simulink library "pixhawk_slib_sensors_actuators"  (R2017b)
settings: Solver=ode45  StartTime=0.0  StopTime=10.0  RelTol=1e-3
undefined symbols (not defined in the file): PixhawkBlock_InitFcn
libraries: pixhawk_slib_uORB_RW x6
settings Model: Creator=skuznick  LastModifiedBy=uavcs
settings DataIOCC: LimitDataPoints=on  SaveFormat=Array
settings OptimizationCC: BlockReduction=off  BooleanDataType=off  LifeSpan=inf
settings DebuggingCC: SaveWithParameterizedLinksMsg=none  UnderspecifiedInitializationDetection=Classic  MergeDetectMultiDrivingBlocksExec=none  SignalResolutionControl=TryResolveAllWithWarning  AllowSymbolicDim=off  StrictBusMsg=Warning  SFUnexpectedBacktrackingDiag=warning  SFNoUnconditionalDefaultTransitionDiag=warning  SFExecutionAtInitializationDiag=none
settings HardwareCC: ProdBitPerPointer=32  ProdBitPerSizeT=32  ProdBitPerPtrDiffT=32  ProdLargestAtomicFloat=None  ProdIntDivRoundTo=Undefined  ProdEndianess=Unspecified  ProdWordSize=32  ProdHWDeviceType=32-bit Generic  TargetUnknown=on
settings ModelReferenceCC: PropagateSignalLabelsOutOfModel=off
settings CodeAppCC: StateflowObjectComments=on
settings GRTTargetCC: TargetLangStandard=C89/C90 (ANSI)  GeneratePreprocessorConditionals=Disable all
settings ConfigComp: CovMetricSettings=dw  CovHtmlReporting=on  CovSaveCumulativeToWorkspaceVar=on  CovSaveSingleToWorkspaceVar=on  CovExternalEMLEnable=off  CovSFcnEnable=off

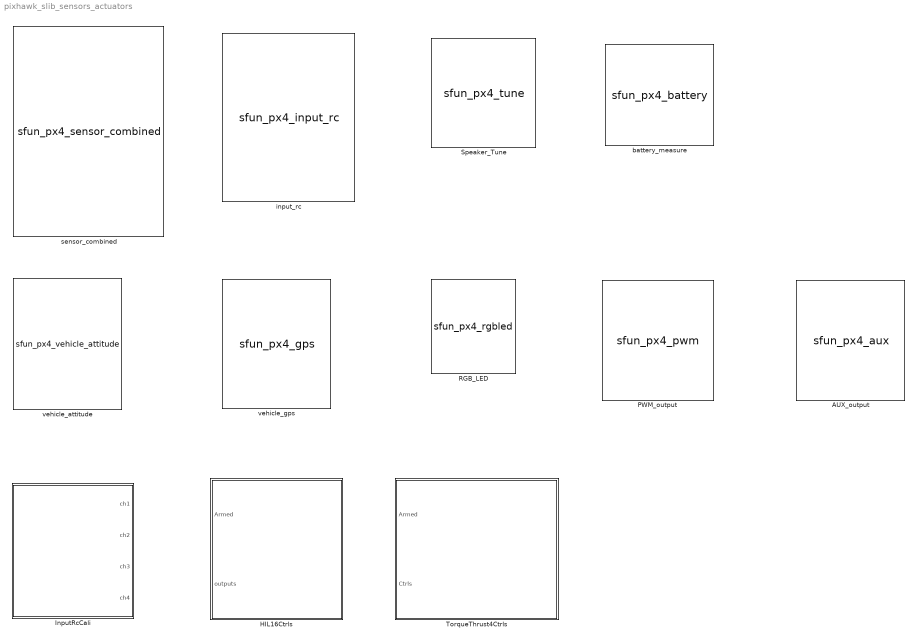
== system pixhawk_slib_sensors_actuators ==
  AUX_output : S-Function  Description=|  InitFcn=|  FunctionName=sfun_px4_aux  Parameters=show_aux1,show_aux2,show_aux3,show_aux4,show_aux5,show_aux6,pwm_rate  SFunctionDeploymentMode=off  EnableBusSupport=off  mask(PX4_Output_AUX){pwm_rate=400Hz, show_aux1=on, show_aux4=off, show_aux2=on, show_aux5=off, show_aux3=off, show_aux6=off}
      Description=|
      | This block allows the user to send the appropriate PWM signals out to the PX4 AUX outputs.  
      | These are usually connected to the ESCs which control the motor speeds. 
      | In order for the flight control to arm (enable) the output from the software side, the ARM Output input must be held high (boolean TRUE).  
      | Only then will the PWM values be sent out the PX4 hardware ports.  
      | This is usually a function of the RC Tx in combination with other flight modes programmed in the Simulink model by the user.  
      | The block has 8 available ports (data type uint16) which can be selectively chosen.  
      | These correspond to the 6 PWM (optional on 5/6) output ports on the px4fmu hardware. 
      | 
      | You *must* ensure that the line: “fmu mode_pwm” appears in your rc.txt file or manually run this from a Nuttx terminal *before* you start the px4_simulink_app module.  
      | Also – note: the FMU only has to be ARMED for the AUX pins to work – the Hardware safety switch is only for the IO.  
      | The switch’s blink code tells you what is armed.  You have to ARM both the Hardware switch and Software block in order to get the PWM output to work, but only the Software block for the AUX outputs.
      InitFcn=|
      | PixhawkBlock_InitFcn;
      | codertarget.pixhawk.blocks.Block_Callbacks.checkSingleInstance(gcb);
      mask prompts: pwm_rate "PWM Update Rate"; show_aux1 "AUX 1"; show_aux4 "AUX 4"; show_aux2 "AUX 2"; show_aux5 "AUX 5"; show_aux3 "AUX 3"; show_aux6 "AUX 6"
      mask help:
      | AUX PWM Output Block
      |
      | Sends the PWM signals to the output ports of the FMU (Auxillary Ports)
      mask init:
      | show_aux1 = boolean(show_aux1);
      | show_aux2 = boolean(show_aux2);
      | show_aux3 = boolean(show_aux3);
      | show_aux4 = boolean(show_aux4);
      | show_aux5 = boolean(show_aux5);
      | show_aux6 = boolean(show_aux6);
      mask Help: eval('sharedhelp(''AUX_output'')');
      mask TypeOptions pwm_rate: 50Hz | 125Hz | 250Hz | 300Hz | 400Hz
      mask DialogControl Container2 Prompt: Output PWM AUX Selection
      mask Display:
      | image('mask_aux.jpg');
      | port_label('input',1,'ARM Output');
      | idx = 2;
      | show_port = get_param(gcb,'show_aux1');
      | if strcmp(show_port,'on') == true
      |     port_label('input',idx,'aux1');
      |     idx = idx + 1;
      | end
      | show_port = get_param(gcb,'show_aux2');
      | if strcmp(show_port,'on') == true
      |     port_label('input',idx,'aux2');
      |     idx = idx + 1;
      | end
      | show_port = get_param(gcb,'show_aux3');
      | if strcmp(show_port,'on') == true
      |     port_label('input',idx,'aux3');
      |     idx = idx + 1;
      | end
      | show_port = get_param(gcb,'show_aux4');
      | if strcmp(show_port,'on') == true
      |     port_label('input',idx,'aux4');
      |     idx = idx + 1;
      | end
      | show_port = get_param(gcb,'show_aux5');
      | if strcmp(show_port,'on') == true
      |     port_label('input',idx,'aux5');
      |     idx = idx + 1;
      | end
      | show_port = get_param(gcb,'show_aux6');
      | if strcmp(show_port,'on') == true
      |     port_label('input',idx,'aux6');
      | end
  HIL16Ctrls : Subsystem
      mask Help: eval('sharedhelp(''HIL16CtrlsPWM'')');
      mask DialogControl Control2 Prompt: This block gets 16D control signals for HIL simulation with range from 1000 to 2000
      mask Display:
      | fprintf('Controls for HIL \n 1D Arm: 0 or 1 \n 16D Ctrls: 1000 to 2000 ')
      | 
      | port_label('input', 1, 'Arm');
      | port_label('input', 2, 'Ctrls');
  InputRcCali : Subsystem
      mask Help: eval('sharedhelp(''InputRcCali'')');
      mask DialogControl Control2 Prompt: This block outputs cablibrated RC pwms for ch1 to ch4 with range 1100 to 1900
      mask Display:
      | fprintf('Calibrated RC PWMs \n CH1-CH4: 1100 to 1900 ')
      | 
      | port_label('output', 1, 'ch1');
      | port_label('output', 2, 'ch2');
      | port_label('output', 3, 'ch3');
      | port_label('output', 4, 'ch4');
  PWM_output : S-Function  Description=|  InitFcn=|  FunctionName=sfun_px4_pwm  Parameters=show_pwm1,show_pwm2,show_pwm3,show_pwm4,show_pwm5,show_pwm6,show_pwm7,show_pwm8,pwm_rate,pub_outputs  SFunctionDeploymentMode=off  EnableBusSupport=off  mask(PX4_Output_PWM){pub_outputs=on, pwm_rate=400Hz, show_pwm1=on, show_pwm5=off, show_pwm2=on, show_pwm6=off, show_pwm3=on, show_pwm7=off, show_pwm4=on, show_pwm8=off}
      Description=|
      | This block allows the user to send the appropriate PWM signals out to the PX4 outputs.  
      | These are usually connected to the ESCs which control the motor speeds. 
      | In order for the flight control to arm (enable) the output from the software side, the ARM Output input must be held high (boolean TRUE).  
      | Only then will the PWM values be sent out the PX4 hardware ports.  
      | This is usually a function of the RC Tx in combination with other flight modes programmed in the Simulink model by the user.  
      | The block has 8 available ports (data type uint16) which can be selectively chosen.  
      | These correspond to the 8 PWM output ports on the px4fmu hardware.
      InitFcn=|
      | PixhawkBlock_InitFcn;
      | codertarget.pixhawk.blocks.Block_Callbacks.checkSingleInstance(gcb);
      mask prompts: pub_outputs "Publish Outputs (actuator_outputs)"; pwm_rate "PWM Update Rate"; show_pwm1 "PWM 1"; show_pwm5 "PWM 5"; show_pwm2 "PWM 2"; show_pwm6 "PWM 6"; show_pwm3 "PWM 3"; show_pwm7 "PWM 7"; show_pwm4 "PWM 4"; show_pwm8 "PWM 8"
      mask help:
      | PWM Output Block
      |
      | Sends the PWM signals to the output ports of the PX4IO
      mask init:
      | show_pwm1 = boolean(show_pwm1);
      | show_pwm2 = boolean(show_pwm2);
      | show_pwm3 = boolean(show_pwm3);
      | show_pwm4 = boolean(show_pwm4);
      | show_pwm5 = boolean(show_pwm5);
      | show_pwm6 = boolean(show_pwm6);
      | show_pwm7 = boolean(show_pwm7);
      | show_pwm8 = boolean(show_pwm8);
      | pub_outputs = boolean(pub_outputs);
      mask Help: eval('sharedhelp(''PWM_output'')');
      mask TypeOptions pwm_rate: 50Hz | 125Hz | 250Hz | 300Hz | 400Hz
      mask DialogControl Container2 Prompt: Output PWM Selection
      mask Display:
      | image('mask_pwm.jpg');
      | port_label('input',1,'ARM Output');
      | idx = 2;
      | show_port = get_param(gcb,'show_pwm1');
      | if strcmp(show_port,'on') == true
      |     port_label('input',idx,'pwm1');
      |     idx = idx + 1;
      | end
      | show_port = get_param(gcb,'show_pwm2');
      | if strcmp(show_port,'on') == true
      |     port_label('input',idx,'pwm2');
      |     idx = idx + 1;
      | end
      | show_port = get_param(gcb,'show_pwm3');
      | if strcmp(show_port,'on') == true
      |     port_label('input',idx,'pwm3');
      |     idx = idx + 1;
      | end
      | show_port = get_param(gcb,'show_pwm4');
      | if strcmp(show_port,'on') == true
      |     port_label('input',idx,'pwm4');
      |     idx = idx + 1;
      | end
      | show_port = get_param(gcb,'show_pwm5');
      | if strcmp(show_port,'on') == true
      |     port_label('input',idx,'pwm5');
      |     idx = idx + 1;
      | end
      | show_port = get_param(gcb,'show_pwm6');
      | if strcmp(show_port,'on') == true
      |     port_label('input',idx,'pwm6');
      |     idx = idx + 1;
      | end
      | show_port = get_param(gcb,'show_pwm7');
      | if strcmp(show_port,'on') == true
      |     port_label('input',idx,'pwm7');
      |     idx = idx + 1;
      | end
      | show_port = get_param(gcb,'show_pwm8');
      | if strcmp(show_port,'on') == true
      |     port_label('input',idx,'pwm8');
      |     idx = idx + 1;
      | end
  RGB_LED : S-Function  Description=|  InitFcn=PixhawkBlock_InitFcn;  FunctionName=sfun_px4_rgbled  SFunctionDeploymentMode=off  EnableBusSupport=off  SFcnStateName=sl_led_control_s  mask(PX4_RGBLED - controls the mode and color of the Pixhawk RGB LED){}
      | This block gives the user control over various lighting modes of the RGB LED available on the PX4 hardware. 
      | This block accepts 2 inputs: Mode and Color.  These are enumeration data types.  You can find out what values are valid in the MATLAB command window by typing: 
      | Enumeration members for class 'RGBLED_COLOR_ENUM':
      |     SL_COLOR_OFF
      |     SL_COLOR_RED
      |     SL_COLOR_GREEN
      |     SL_COLOR_BLUE
      |     SL_COLOR_YELLOW
      |     SL_COLOR_PURPLE
      |     SL_COLOR_AMBER
      |     SL_COLOR_CYAN
      |     SL_COLOR_WHITE 
      | Enumeration members for class 'RGBLED_MODE_ENUM':
      |     SL_MODE_OFF
      |     SL_MODE_ON
      |     SL_MODE_DISABLED
      |     SL_MODE_BLINK_SLOW
      |     SL_MODE_BLINK_NORMAL
      |     SL_MODE_BLINK_FAST
      |     SL_MODE_BREATHE  
      | Look at the sample Simulink model: px4demo_rgbled.slx for an example of how to use this block.
      mask help:
      | LED Output Block
      |
      | Blocks has input for controlling the Mode and Color of the RGB LED light on the pixhawk.
      settings: SFcnIsStateOwnerBlock=on
      mask Help: eval('sharedhelp(''RGB_LED'')');
      mask Display:
      | image('mask_rgbled.jpg');
      | port_label('input',1,'Mode');
      | port_label('input',2,'Color');
  Speaker_Tune : S-Function  InitFcn=PixhawkBlock_InitFcn;  FunctionName=sfun_px4_tune  SFunctionDeploymentMode=off  EnableBusSupport=off  SFcnStateName=tune_msg  mask(PX4_Play_Tune - Plays a predefined tune or one based on a "string"){}
      mask help:
      | Tone Output Block
      |
      | For Tone ID: use one of the PX4_TUNE_ENUM values
      | For IsTuneOverride  input: if set to 1 the tune which is playing will be stopped and the new started
      | For Trigger input: If it changes from 0 to 1, the tune message will be sent, the buzzser will change its voice.
      settings: SFcnIsStateOwnerBlock=on
      mask Help: eval('sharedhelp(''Speaker_Tune'')');
      mask Display:
      | image('mask_tune.jpg')
      | port_label('input',1,'Tune ID')
      | port_label('input',2,'IsTuneOverride');
      | port_label('input',3,'Trigger');
  TorqueThrust4Ctrls : Subsystem
      mask Help: eval('sharedhelp(''TorqueThrustCtrls'')');
      mask DialogControl Control2 Prompt: This block gets the xyz torque and thrust controls with range -1 to 1
      mask Display:
      | fprintf('Torque and Thrust \n Normalized xyz+T \n 1D Arm: 0 or 1 \n 4D Ctrls: -1 to 1 ')
      | 
      | port_label('input', 1, 'Arm');
      | port_label('input', 2, 'Ctrls');
  battery_measure : S-Function  Description=|  FunctionName=sfun_px4_battery  Parameters=SampleTime,boolean(TimeStamp),boolean(VoltageOut),boolean(VoltageFilteredOut),boolean(CurrentOut),boolean(mAH_Out)  SFunctionDeploymentMode=off  EnableBusSupport=off  SFcnStateName=battery_fd  mask(PX4_Battery){SampleTime=1/250, VoltageOut=on, VoltageFilteredOut=off, CurrentOut=on, mAH_Out=on, TimeStamp=on}
      | This block allows the user to monitor the health of the connected battery.  It returns battery level measurements from the uORB topic publisher “battery_status”.
      | 
      | The user has the ability to choose which telemetry data are available as outputs from this block. 
      |   
      | Signal definitions: 
      | Voltage – (single) Battery voltage in volts 
      | Filtered Voltage – (single)  Filtered battery voltage in volts 
      | Current – (single) Battery current in amperes 
      | mAH – (single) Discharged amount in mAh 
      | Timestamp– (int32) timestamp of measurement
      mask prompts: SampleTime "Sample Time"; VoltageOut "Voltage"; VoltageFilteredOut "Filtered Voltage"; CurrentOut "Current"; mAH_Out "mAH"; TimeStamp "Time Stamp"
      mask help:
      | Battery Input Block
      |
      | Provides Battery telemetry data from the Pixhawk hardware
      mask init:
      | VoltageOut = boolean(VoltageOut);
      | VoltageFilteredOut = boolean(VoltageFilteredOut);
      | CurrentOut = boolean(CurrentOut);
      | mAH_Out = boolean(mAH_Out);
      | TimeStamp = boolean(TimeStamp);
      settings: SFcnIsStateOwnerBlock=on
      mask Help: eval('sharedhelp(''battery_measure'')');
      mask DialogControl DescGroupVar Prompt: PX4_Battery_Measurement
      mask DialogControl DescTextVar Prompt: Returns battery measurements from Pixhawk hardware
      mask Display:
      | PortNum = 1;
      | %
      | image('mask_battery.jpg');
      | if TimeStamp>0
      | port_label('output',PortNum,'TimeStamp')
      | PortNum = PortNum + 1;
      | end
      | 
      | if VoltageOut>0
      | port_label('output',PortNum,'Voltage')
      | PortNum = PortNum + 1;
      | end
      | 
      | if VoltageFilteredOut>0
      | port_label('output',PortNum,'Filtered Voltage')
      | PortNum = PortNum + 1;
      | end
      | 
      | if CurrentOut>0
      | port_label('output',PortNum,'Current')
      | PortNum = PortNum + 1;
      | end
      | 
      | if mAH_Out>0
      | port_label('output',PortNum,'mAH')
      | PortNum = PortNum + 1;
      | end
  input_rc : S-Function  Description=|  InitFcn=PixhawkBlock_InitFcn;  FunctionName=sfun_px4_input_rc  Parameters=sampletime,channel1,channel2,channel3,channel4,channel5,channel6,channel7,channel8,channel9,channel10,channel11,channel12,channel13,channel14,channel15,channel16,channel17,channel18,ch_count,rssi,rc_failsafe,rc_lost,rc_inputsource,  SFunctionDeploymentMode=off  EnableBusSupport=off  SFcnStateName=input_rc_fd  mask(PX4_Input_RC){sampletime=1/250, channel1=on, channel2=on, channel3=on, channel4=on, channel5=off, channel6=off, channel7=off, channel8=off, channel9=off, channel10=off, channel11=off, channel12=off, channel13=off, channel14=off, channel15=off, channel16=off, channel17=off, channel18=off, ch_count=off, rssi=off, rc_failsafe=off, rc_lost=off, rc_inputsource=off}
      | RC Input Block
      | 
      | This block provides user input control to the model.
      | It uses the input_rc uORB topic.
      | 
      | The user has the ability to choose which channels are available as outputs from this block and also some optional outputs. These include 
      | Channels 1 through 18
      | double data type indicating the PWM value from the controller 
      | measured pulse widths for each of the supported channels 
      | Channel Count 
      | uint32 data type of the number of channels which are detector by the PX4 
      | RC Failsafe 
      | boolean data types indicating that the RC Tx is sending the FailSafe signal (if equipped and properly setup) 
      | explicit failsafe flag: true on TX failure or TX out of range , false otherwise. 
      | Only the true state is reliable, as there are some (PPM) receivers on the market going into failsafe without telling us explicitly. 
      | RC Input Source 
      | Enumeration data type indicating which source the RC input is from. 
      | Valid values are found in the ENUM file: RC_INPUT_SOURCE_ENUM.m 
      |           Enumeration members for class 'RC_INPUT_SOURCE_ENUM':
      |           RCINPUT_SOURCE_UNKNOWN         (0)
      |           RCINPUT_SOURCE_PX4FMU_PPM      (1)
      |           RCINPUT_SOURCE_PX4IO_PPM       (2)
      |           RCINPUT_SOURCE_PX4IO_SPEKTRUM  (3)
      |           RCINPUT_SOURCE_PX4IO_SBUS      (4)
      |           RCINPUT_SOURCE_PX4IO_ST24      (5)
      |           RCINPUT_SOURCE_MAVLINK         (6)
      |           RCINPUT_SOURCE_QURT            (7)
      |           RCINPUT_SOURCE_PX4FMU_SPEKTRUM (8)
      |           RCINPUT_SOURCE_PX4FMU_SBUS     (9)
      |           RCINPUT_SOURCE_PX4FMU_ST24     (10)
      |           RCINPUT_SOURCE_PX4FMU_SUMD     (11)
      |           RCINPUT_SOURCE_PX4FMU_DSM      (12)
      |           RCINPUT_SOURCE_PX4IO_SUMD      (13)
      | 
      | RSSI - Receive signal strength index 
      | receive signal strength indicator (RSSI): < 0: Undefined, 0: no signal, 255: full reception 
      | RC Lost Connection 
      | boolean data type indicating RC receiver connection status 
      | True, if no frame has arrived in the expected time, false otherwise. 
      | True usally means that the receiver has been disconnected, but can also indicate a radio link loss on "stupid" systems. 
      | Will remain false, if a RX with failsafe option continues to transmit frames after a link loss. 
      |   
      | Sample Model: px4demo_input_rc.slx
      mask prompts: sampletime "Sample Time"; channel1 "Channel 1"; channel2 "Channel 2"; channel3 "Channel 3"; channel4 "Channel 4"; channel5 "Channel 5"; channel6 "Channel 6"; channel7 "Channel 7"; channel8 "Channel 8"; ch_count "Channel Count"; rc_failsafe "RC Failsafe"; rc_lost "RC Lost Connection"; rc_inputsource "RC Input Source"
      mask help:
      | RC Input Block
      |
      | Receiver Inputs from the Pixhawk hardware
      mask init:
      | channel1 = boolean(channel1);
      | channel2 = boolean(channel2);
      | channel3 = boolean(channel3);
      | channel4 = boolean(channel4);
      | channel5 = boolean(channel5);
      | channel6 = boolean(channel6);
      | channel7 = boolean(channel7);
      | channel8 = boolean(channel8);
      | channel9 = boolean(channel9);
      | channel10 = boolean(channel10);
      | channel11 = boolean(channel11);
      | channel12 = boolean(channel12);
      | channel13 = boolean(channel13);
      | channel14 = boolean(channel14);
      | channel15 = boolean(channel15);
      | channel16 = boolean(channel16);
      | channel17 = boolean(channel17);
      | channel18 = boolean(channel18);
      | ch_count = boolean(ch_count);
      | rssi = boolean(rssi);
      | rc_failsafe = boolean(rc_failsafe);
      | rc_lost = boolean(rc_lost);
      | rc_inputsource = boolean(rc_inputsource);
      settings: SFcnIsStateOwnerBlock=on
      mask Help: eval('sharedhelp(''input_rc'')');
      mask DialogControl channelselection Prompt: Channel Selection
      mask DialogControl Container3 Prompt: Optional Outputs
      mask Display:
      | idx = 1;
      | image('mask_input_rc.jpg');
      | show_port = get_param(gcb,'channel1');
      | if strcmp(show_port,'on') == true
      |     port_label('output', idx, 'Ch1');
      |     idx = idx + 1;
      | end
      | show_port = get_param(gcb,'channel2');
      | if strcmp(show_port,'on') == true
      |     port_label('output', idx, 'Ch2');
      |     idx = idx + 1;
      | end
      | show_port = get_param(gcb,'channel3');
      | if strcmp(show_port,'on') == true
      |     port_label('output', idx, 'Ch3');
      |     idx = idx + 1;
      | end
      | show_port = get_param(gcb,'channel4');
      | if strcmp(show_port,'on') == true
      |     port_label('output', idx, 'Ch4');
      |     idx = idx + 1;
      | end
      | show_port = get_param(gcb,'channel5');
      | if strcmp(show_port,'on') == true
      |     port_label('output', idx, 'Ch5');
      |     idx = idx + 1;
      | end
      | show_port = get_param(gcb,'channel6');
      | if strcmp(show_port,'on') == true
      |     port_label('output', idx, 'Ch6');
      |     idx = idx + 1;
      | end
      | show_port = get_param(gcb,'channel7');
      | if strcmp(show_port,'on') == true
      |     port_label('output', idx, 'Ch7');
      |     idx = idx + 1;
      | end
      | show_port = get_param(gcb,'channel8');
      | if strcmp(show_port,'on') == true
      |     port_label('output', idx, 'Ch8');
      |     idx = idx + 1;
      | end
      | show_port = get_param(gcb,'channel9');
      | if strcmp(show_port,'on') == true
      |     port_label('output', idx, 'Ch9');
      |     idx = idx + 1;
      | end
      | show_port = get_param(gcb,'channel10');
      | if strcmp(show_port,'on') == true
      |     port_label('output', idx, 'Ch10');
      |     idx = idx + 1;
      | end
      | show_port = get_param(gcb,'channel11');
      | if strcmp(show_port,'on') == true
      |     port_label('output', idx, 'Ch11');
      |     idx = idx + 1;
      | end
      | show_port = get_param(gcb,'channel12');
      | if strcmp(show_port,'on') == true
      |     port_label('output', idx, 'Ch12');
      |     idx = idx + 1;
      | end
      | show_port = get_param(gcb,'channel13');
      | if strcmp(show_port,'on') == true
      |     port_label('output', idx, 'Ch13');
      |     idx = idx + 1;
      | end
      | show_port = get_param(gcb,'channel14');
      | if strcmp(show_port,'on') == true
      |     port_label('output', idx, 'Ch14');
      |     idx = idx + 1;
      | end
      | show_port = get_param(gcb,'channel15');
      | if strcmp(show_port,'on') == true
      |     port_label('output', idx, 'Ch15');
      |     idx = idx + 1;
      | end
      | show_port = get_param(gcb,'channel16');
      | if strcmp(show_port,'on') == true
      |     port_label('output', idx, 'Ch16');
      |     idx = idx + 1;
      | end
      | show_port = get_param(gcb,'channel17');
      | if strcmp(show_port,'on') == true
      |     port_label('output', idx, 'Ch17');
      |     idx = idx + 1;
      | end
      | show_port = get_param(gcb,'channel18');
      | if strcmp(show_port,'on') == true
      |     port_label('output', idx, 'Ch18');
      |     idx = idx + 1;
      | end
      | show_port = get_param(gcb,'ch_count');
      | if strcmp(show_port,'on') == true
      |     port_label('output', idx, 'Num Ch');
      |     idx = idx + 1;
      | end
      | show_port = get_param(gcb,'rssi');
      | if strcmp(show_port,'on') == true
      |     port_label('output', idx, 'RSSI');
      |     idx = idx + 1;
      | end
      | show_port = get_param(gcb,'rc_failsafe');
      | if strcmp(show_port,'on') == true
      |     port_label('output', idx, 'RC Failsafe');
      |     idx = idx + 1;
      | end
      | show_port = get_param(gcb,'rc_lost');
      | if strcmp(show_port,'on') == true
      |     port_label('output', idx, 'RC Lost');
      |     idx = idx + 1;
      | end
      | show_port = get_param(gcb,'rc_inputsource');
      | if strcmp(show_port,'on') == true
      |     port_label('output', idx, 'RC Source');
      |     idx = idx + 1;
      | end
  sensor_combined : S-Function  Description=|  InitFcn=PixhawkBlock_InitFcn;  FunctionName=sfun_px4_sensor_combined  Parameters=sampletime, show_mag, show_acc, show_gyro, show_baro, show_ts  SFunctionDeploymentMode=off  EnableBusSupport=off  SFcnStateName=sensor_fd  mask(PX4_Sensor_Combined){sampletime=1/250, show_mag=on, show_acc=on, show_gyro=on, show_baro=on, show_ts=on}
      | Sensor Combined Block
      | 
      | This block enables access to the various sensors available on the px4fmu-v2 hardware.  
      | The user can use these signals in the Simulink control model.  
      | The sample time needs to be provided in the mask dialog.  
      | Optional output ports can also be selected.  
      | Refer to the sample model: px4demo_attitude_control.slx
      | 
      | Signal definitions: 
      | Magnetometer (x,y,z) - single values – Magnetic field in NED body frame, in Gauss 
      | Accelerometer (x,y,z) - single values – Acceleration in NED body frame, in m/s^2 
      | Gyroscope (p,q,r) - single values – Angular velocity in radians per second 
      | Barometer (Altitude) - single value – Barometric pressure, already temperature compensated (millibars) 
      | RunTime (timestamp) - double value – Timestamp in microseconds since boot, from gyro 
      |   
      | The sensor_combined block needs to have the px4io service running on the PX4 hardware in order to get valid signal values.
      mask prompts: sampletime "Sample Time"; show_mag "Magnetometer (x,y,z)"; show_acc "Accelerometer (x,y,z)"; show_gyro "Gyroscope (x,y,z)"; show_baro "Barometer (Altitude)"; show_ts "uORB and RunTime (timestamp)"
      mask help:
      | Sensor Input Block
      |
      | Sensor Combined inputs from the Pixhawk hardware
      mask init:
      | show_mag = boolean(show_mag);
      | show_acc = boolean(show_acc);
      | show_gyro = boolean(show_gyro);
      | show_baro = boolean(show_baro);
      | show_ts = boolean(show_ts);
      settings: SFcnIsStateOwnerBlock=on
      mask Help: eval('sharedhelp(''sensor_combined'')');
      mask DialogControl Container2 Prompt: Output Selection
      mask Display:
      | idx = 1;
      | image('mask_sensor_combined.jpg');
      | show_port = get_param(gcb,'show_mag');
      | if strcmp(show_port,'on') == true
      |     port_label('output', idx, 'MagX');
      |     idx = idx + 1;
      |     port_label('output', idx, 'MagY');
      |     idx = idx + 1;
      |     port_label('output', idx, 'MagZ');
      |     idx = idx + 1;
      | end
      | 
      | show_port = get_param(gcb,'show_acc');
      | if strcmp(show_port,'on') == true
      |     port_label('output', idx, 'AccelX');
      |     idx = idx + 1;
      |     port_label('output', idx, 'AccelY');
      |     idx = idx + 1;
      |     port_label('output', idx, 'AccelZ');
      |     idx = idx + 1;
      | end
      | 
      | show_port = get_param(gcb,'show_gyro');
      | if strcmp(show_port,'on') == true
      |     port_label('output', idx, 'GyroX (p)');
      |     idx = idx + 1;
      |     port_label('output', idx, 'GyroY (q)');
      |     idx = idx + 1;
      |     port_label('output', idx, 'GyroZ (r)');
      |     idx = idx + 1;
      | end
      | 
      | show_port = get_param(gcb,'show_baro');
      | if strcmp(show_port,'on') == true
      |     port_label('output', idx, 'Baro');
      |     idx = idx + 1;
      | end
      | 
      | show_port = get_param(gcb,'show_ts');
      | if strcmp(show_port,'on') == true
      |     port_label('output', idx, 'Mag Ts')
      |     idx = idx + 1;
      |     port_label('output', idx, 'Accel Ts')
      |     idx = idx + 1;
      |     port_label('output', idx, 'Baro Ts')
      |     idx = idx + 1;
      |     port_label('output', idx, 'uORB Ts')
      | 
      | end
  vehicle_attitude : S-Function  Description=|  InitFcn=PixhawkBlock_InitFcn;  FunctionName=sfun_px4_vehicle_attitude  Parameters=sampletime, show_r, show_p, show_y, show_q,show_ts  SFunctionDeploymentMode=off  EnableBusSupport=off  SFcnStateName=angeuler_fd  mask(PX4_Vehicle_Attitude){sampletime=0.01, show_r=on, show_p=on, show_y=on, show_q=on, show_ts=on}
      | This block gives access to the running service that calculates the vehicle’s attitude.  A uORB topic (vehicle_attitude (attitude measurements)) publisher MUST be running in order for this block to provide valid signal values.  The available ones as of v1.3 are: 
      | attitude_estimator_ekf – EKF-Extended Kalman Filter for attitude estimation 
      | attitude_estimator_so3 – SO(3)-attitude estimation by using accelerometer, gyroscopes and magnetometer 
      | One of these MUST be running on the px4fmu in order for this block to return valid values.  Refer to the sample model: px4demo_attitude_control.slx. Attitude in NED (North-East-Down) body frame in SI units. 
      | Signal definitions: 
      | Roll – single value, Roll angle (rad, Tait-Bryan, NED) 
      | Pitch – single value, Pitch angle (rad, Tait-Bryan, NED) 
      | Yaw – single value, Yaw angle (rad, Tait-Bryan, NED) 
      | Quaternion (NED) – single(4) values (optional based on the uORB publisher)
      mask prompts: sampletime "Sample Time"; show_r "Roll rate"; show_p "Pitch rate"; show_y "Yaw rate"; show_q "Quaternion (NED)"; show_ts "uORB Ts"
      mask help:
      | Vehicle Attitude  Block
      |
      | Vehicle Attitude measurements from the Pixhawk hardware
      mask init:
      | show_r = boolean(show_r);
      | show_p = boolean(show_p);
      | show_y = boolean(show_y);
      | show_q = boolean(show_q);
      | show_ts = boolean(show_ts);
      settings: SFcnIsStateOwnerBlock=on
      mask Help: eval('sharedhelp(''vehicle_attitude'')');
      mask DialogControl Container2 Prompt: Output Signal Selection
      mask Display:
      | idx = 1;
      | image('mask_vehicle_attitude.jpg');
      | show_port = get_param(gcb,'show_r');
      | if strcmp(show_port,'on') == true
      |     port_label('output', idx, 'Roll rate (phi)');
      |     idx = idx + 1;
      | end
      | show_port = get_param(gcb,'show_p');
      | if strcmp(show_port,'on') == true
      |     port_label('output', idx, 'Pitch rate (theta)');
      |     idx = idx + 1;
      | end
      | show_port = get_param(gcb,'show_y');
      | if strcmp(show_port,'on') == true
      |     port_label('output', idx, 'Yaw rate (psi)');
      |     idx = idx + 1;
      | end
      | show_port = get_param(gcb,'show_q');
      | if strcmp(show_port,'on') == true
      |     port_label('output', idx, 'Quaternion');
      |     idx = idx + 1;
      | end
      | show_port = get_param(gcb,'show_ts');
      | if strcmp(show_port,'on') == true
      |     port_label('output', idx, 'uORB TS');
      |     idx = idx + 1;
      | end
  vehicle_gps : S-Function  Description=|  FunctionName=sfun_px4_gps  Parameters=sampletime, show_alt, show_ts_gps, show_vel, show_fixtype, show_numsat  SFunctionDeploymentMode=off  EnableBusSupport=off  SFcnStateName=gps_fd  mask(PX4_Vehicle_GPS){sampletime=1/250, show_alt=on, show_ts_gps=on, show_vel=on, show_fixtype=on, show_numsat=on}
      | This block will provide GPS signals from the uORB topic publisher: vehicle_gps_position.  
      | You must ensure that you have the gps topic executed as part of the start-up script in order to get valid signal values. 
      | Refer to the sample model: px4demo_gps.slx 
      | Signal definitions: 
      | Latitude – (int32) global coordinate given in 1e-7 degrees 
      | Longitude – (int32) global coordinate given in 1e-7 degrees 
      | Position TS – (double) timestamp for position information 
      | Altitude – (int32) in 1e-3 meters (millimeters) above MSL (mean sea level) 
      | GPS TS – (double) timestamp (microseconds in GPS format).  This is the timestamp that comes from the GPS module. 
      | Velocity TS – (single) timestamp for velocity information 
      | Velocity – (single) GPS ground speed in meters/second 
      | GPS Fix Type – (uint8) 0-1 = No fix, 2 = 2D fix, 3= 3D fix 
      | Num Satellites – (uint8) the number of satellites used in calculations
      mask prompts: sampletime "Sample Time"; show_alt "Altitude"; show_ts_gps "GPS Timestamp"; show_vel "Velocity"; show_fixtype "Fix Type"; show_numsat "Number of Satellites"
      mask help:
      | GPS Input Block
      |
      | Return Values from the GPS topic running on the Pixhawk.
      mask init:
      | %show_ts_pos = boolean(show_ts_pos);
      | show_alt = boolean(show_alt);
      | show_ts_gps = boolean(show_ts_gps);
      | show_vel = boolean(show_vel);
      | show_fixtype = boolean(show_fixtype);
      | show_numsat = boolean(show_numsat);
      settings: SFcnIsStateOwnerBlock=on
      mask Help: eval('sharedhelp(''vehicle_gps'')');
      mask DialogControl Container Prompt: Output Selection
      mask Display:
      | idx = 1;
      | image('mask_gps.jpg');
      | port_label('output', idx, 'Latitude');
      | idx = idx + 1;
      | port_label('output', idx, 'Longitude');
      | idx = idx + 1;
      | 
      | % show_port = get_param(gcb,'show_ts_pos');
      | % if strcmp(show_port,'on') == true
      | %     port_label('output', idx, 'Position TS');
      | %     idx = idx + 1;
      | % end
      | 
      | show_port = get_param(gcb,'show_alt');
      | if strcmp(show_port,'on') == true
      |     port_label('output', idx, 'Altitude');
      |     idx = idx + 1;
      | end
      | show_port = get_param(gcb,'show_ts_gps');
      | if strcmp(show_port,'on') == true
      |     port_label('output', idx, 'GPS TS');
      |     idx = idx + 1;
      | end
      | show_port = get_param(gcb,'show_vel');
      | if strcmp(show_port,'on') == true
      |    % port_label('output', idx, 'Velocity TS');
      |    % idx = idx + 1;
      |     port_label('output', idx, 'Velocity');
      |     idx = idx + 1;
      | end
      | show_port = get_param(gcb,'show_fixtype');
      | if strcmp(show_port,'on') == true
      |     port_label('output', idx, 'GPS Fix Type');
      |     idx = idx + 1;
      | end
      | show_port = get_param(gcb,'show_numsat');
      | if strcmp(show_port,'on') == true
      |     port_label('output', idx, 'Num Satellites');
      |     idx = idx + 1;
      | end

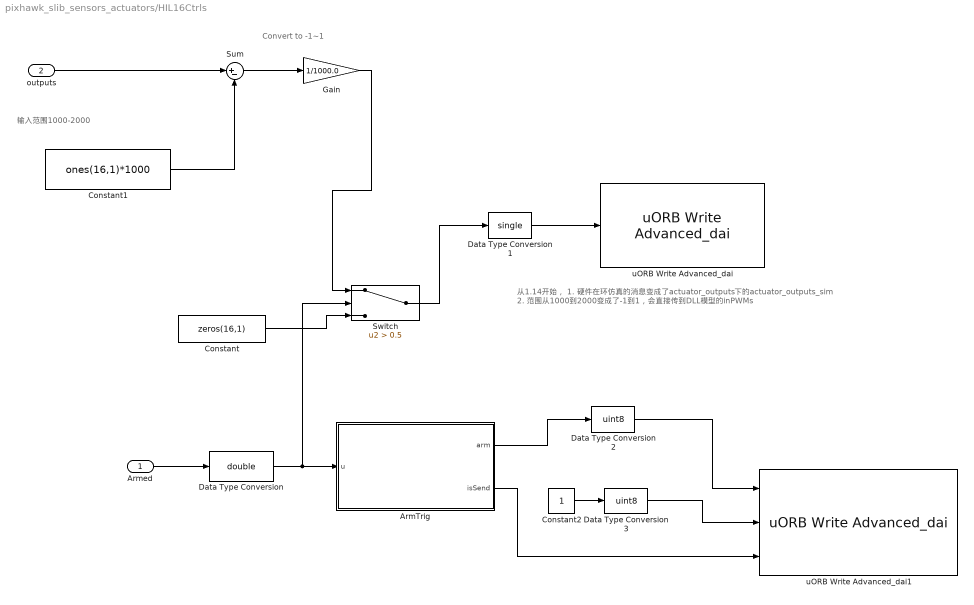
== system pixhawk_slib_sensors_actuators/HIL16Ctrls ==
  note: 从1.14开始，
      | 1. 硬件在环仿真的消息变成了actuator_outputs下的actuator_outputs_sim
      | 2. 范围从1000到2000变成了-1到1，会直接传到DLL模型的inPWMs
  note: 输入范围1000-2000
  note: Convert to -1~1
  Armed : Inport  PortDimensions=1
  outputs : Inport  Port=2  PortDimensions=16
  ArmTrig : MATLAB Function  TreatAsAtomicUnit=on
  Constant : Constant  Value=zeros(16,1)
  Constant1 : Constant  Value=ones(16,1)*1000
  Constant2 : Constant
  Data Type Conversion : DataTypeConversion  OutDataTypeStr=double
  Data Type Conversion1 : DataTypeConversion  OutDataTypeStr=single
  Data Type Conversion2 : DataTypeConversion  OutDataTypeStr=uint8
  Data Type Conversion3 : DataTypeConversion  OutDataTypeStr=uint8
  Gain : Gain  Gain=1/1000.0
  Sum : Sum  Inputs=|+-
  Switch : Switch  Criteria=u2 > Threshold  Threshold=0.5
  uORB Write Advanced_dai : pixhawk_slib_uORB_RW/uORB Write Advanced_dai  Ts=0  uORB_AdvtQueue=on  uORB_FieldEnabledArr="0  0  0  1  0  0  0  0  0  0  0"  uORB_Topic_str=0  uORB_Topic_str_ID=0  uORB_Struct_DT="[1  1  1  1  1]"  BlockInputCount=5  uORB_StructParams="[\"voltage_v\",\"voltage_filtered_v\",\"current_a\",\"current_filtered_a\",\"remaining\"]"  uORB_PortSizes="[1  1  1  1]"  MsgSizeOf=0  MW_update=true
      settings: SourceProductName=Pixhawk Target Blocks
  uORB Write Advanced_dai1 : pixhawk_slib_uORB_RW/uORB Write Advanced_dai  Ts=0  uORB_AdvtQueue=on  uORB_FieldEnabledArr="0  0  0  1  0  0  0  0  0  0  0"  uORB_Topic_str=0  uORB_Topic_str_ID=0  uORB_Struct_DT="[1  1  1  1  1]"  BlockInputCount=5  uORB_StructParams="[\"voltage_v\",\"voltage_filtered_v\",\"current_a\",\"current_filtered_a\",\"remaining\"]"  uORB_PortSizes="[1  1  1  1]"  MsgSizeOf=0  MW_update=true
      settings: SourceProductName=Pixhawk Target Blocks
  wires:
  ArmTrig/2(isSend) -> uORB Write Advanced_dai1/3
  Data Type Conversion2/1 -> uORB Write Advanced_dai1/1
  ArmTrig/1(arm) -> Data Type Conversion2/1
  Constant2/1 -> Data Type Conversion3/1
  Data Type Conversion3/1 -> uORB Write Advanced_dai1/2
  Armed/1 -> Data Type Conversion/1
  Data Type Conversion/1 -> Switch/2, ArmTrig/1(u)
  Data Type Conversion1/1 -> uORB Write Advanced_dai/1
  Constant/1 -> Switch/3
  Switch/1 -> Data Type Conversion1/1
  outputs/1 -> Sum/1
  Constant1/1 -> Sum/2
  Sum/1 -> Gain/1
  Gain/1 -> Switch/1

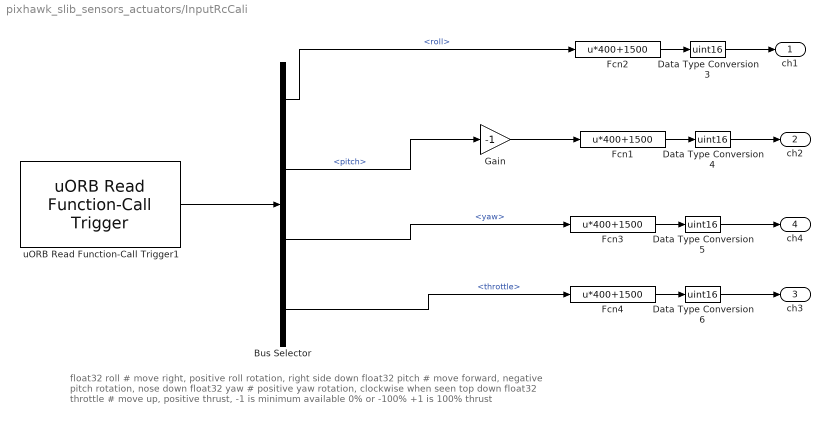
== system pixhawk_slib_sensors_actuators/InputRcCali ==
  note: float32 roll     # move right,   positive roll rotation,  right side down
      | float32 pitch    # move forward, negative pitch rotation, nose down
      | float32 yaw      #               positive yaw rotation,   clockwise when seen top down
      | float32 throttle # move up,      positive thrust,         -1 is minimum available 0% or -100% +1 is 100% thrust
  Bus Selector : BusSelector  OutputSignals=roll,pitch,yaw,throttle
  Data Type Conversion{3..6} (4 alike) : DataTypeConversion  OutDataTypeStr=uint16
  Fcn{1..4} (4 alike) : Fcn  Expr=u*400+1500
  Gain : Gain  Gain=-1
  uORB Read Function-Call Trigger1 : pixhawk_slib_uORB_RW/uORB Read Function-Call Trigger  uORB_Topic_str='manual_control_setpoint'  BusObjVar=Bus: manual_control_setpoint_SL  uORB_Interval=2  AsyncOutput=off  Fcn_call_select=Generate Function Call Signal  TaskName='Task1'  Poll_timeout=-1  Ts=-1
      settings: SourceProductName=Pixhawk Target Blocks
  ch1 : Outport
  ch2 : Outport  Port=2
  ch3 : Outport  Port=3
  ch4 : Outport  Port=4
  wires:
  uORB Read Function-Call Trigger1/1 -> Bus Selector/1
  Gain/1 -> Fcn1/1
  Data Type Conversion3/1 -> ch1/1
  Fcn4/1 -> Data Type Conversion6/1
  Fcn3/1 -> Data Type Conversion5/1
  Data Type Conversion4/1 -> ch2/1
  Data Type Conversion6/1 -> ch3/1
  Fcn1/1 -> Data Type Conversion4/1
  Data Type Conversion5/1 -> ch4/1
  Bus Selector/4 -> Fcn4/1  "<throttle>"
  Bus Selector/2 -> Gain/1  "<pitch>"
  Bus Selector/3 -> Fcn3/1  "<yaw>"
  Fcn2/1 -> Data Type Conversion3/1
  Bus Selector/1 -> Fcn2/1  "<roll>"

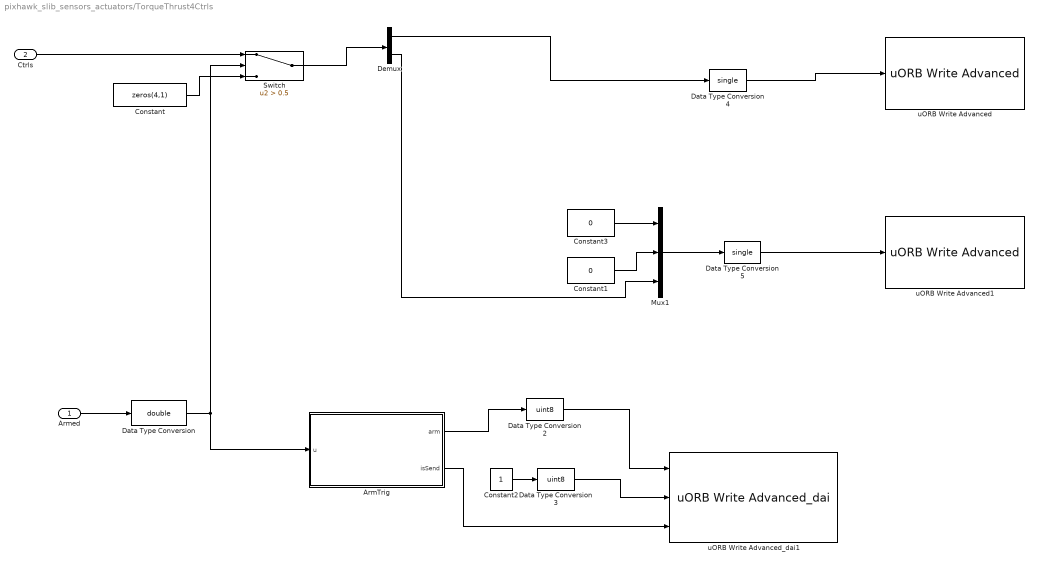
== system pixhawk_slib_sensors_actuators/TorqueThrust4Ctrls ==
  Armed : Inport
  Ctrls : Inport  Port=2  PortDimensions=4
  ArmTrig : MATLAB Function  TreatAsAtomicUnit=on
  Constant : Constant  Value=zeros(4,1)
  Constant1 : Constant  Value=0
  Constant2 : Constant
  Constant3 : Constant  Value=0
  Data Type Conversion : DataTypeConversion  OutDataTypeStr=double
  Data Type Conversion2 : DataTypeConversion  OutDataTypeStr=uint8
  Data Type Conversion3 : DataTypeConversion  OutDataTypeStr=uint8
  Data Type Conversion4 : DataTypeConversion  OutDataTypeStr=single
  Data Type Conversion5 : DataTypeConversion  OutDataTypeStr=single
  Demux : Demux  Outputs=[3,1]
  Mux1 : Mux  Inputs=3
  Switch : Switch  Criteria=u2 > Threshold  Threshold=0.5
  uORB Write Advanced : pixhawk_slib_uORB_RW/uORB Write Advanced  Ts=0  uORB_AdvtQueue=on  uORB_FieldEnabledArr="0  0  0  1  0  0  0  0  0  0  0"  uORB_Topic_str=0  uORB_Struct_DT="[1  1  1  1  1]"  BlockInputCount=5  uORB_StructParams="[\"voltage_v\",\"voltage_filtered_v\",\"current_a\",\"current_filtered_a\",\"remaining\"]"  uORB_PortSizes="[1  1  1  1]"  MsgSizeOf=0  MW_update=true
      settings: SourceProductName=Pixhawk Target Blocks
  uORB Write Advanced1 : pixhawk_slib_uORB_RW/uORB Write Advanced  Ts=0  uORB_AdvtQueue=on  uORB_FieldEnabledArr="0  0  0  1  0  0  0  0  0  0  0"  uORB_Topic_str=0  uORB_Struct_DT="[1  1  1  1  1]"  BlockInputCount=5  uORB_StructParams="[\"voltage_v\",\"voltage_filtered_v\",\"current_a\",\"current_filtered_a\",\"remaining\"]"  uORB_PortSizes="[1  1  1  1]"  MsgSizeOf=0  MW_update=true
      settings: SourceProductName=Pixhawk Target Blocks
  uORB Write Advanced_dai1 : pixhawk_slib_uORB_RW/uORB Write Advanced_dai  Ts=0  uORB_AdvtQueue=on  uORB_FieldEnabledArr="0  0  0  1  0  0  0  0  0  0  0"  uORB_Topic_str=0  uORB_Topic_str_ID=0  uORB_Struct_DT="[1  1  1  1  1]"  BlockInputCount=5  uORB_StructParams="[\"voltage_v\",\"voltage_filtered_v\",\"current_a\",\"current_filtered_a\",\"remaining\"]"  uORB_PortSizes="[1  1  1  1]"  MsgSizeOf=0  MW_update=true
      settings: SourceProductName=Pixhawk Target Blocks
  wires:
  Constant/1 -> Switch/3
  Armed/1 -> Data Type Conversion/1
  Ctrls/1 -> Switch/1
  Data Type Conversion/1 -> ArmTrig/1(u), Switch/2
  Switch/1 -> Demux/1
  Constant3/1 -> Mux1/1
  Constant1/1 -> Mux1/2
  Demux/2 -> Mux1/3
  Mux1/1 -> Data Type Conversion5/1
  Data Type Conversion4/1 -> uORB Write Advanced/1
  Data Type Conversion5/1 -> uORB Write Advanced1/1
  Demux/1 -> Data Type Conversion4/1
  Data Type Conversion3/1 -> uORB Write Advanced_dai1/2
  Data Type Conversion2/1 -> uORB Write Advanced_dai1/1
  Constant2/1 -> Data Type Conversion3/1
  ArmTrig/1(arm) -> Data Type Conversion2/1
  ArmTrig/2(isSend) -> uORB Write Advanced_dai1/3

== matlab function pixhawk_slib_sensors_actuators/HIL16Ctrls/ArmTrig ==
  data: u input; arm output; isSend output
function [arm,isSend] = fcn(u)

persistent lastArm;
if isempty(lastArm)
    lastArm=0;
end

isSend=0;
arm=u;

if abs(arm-lastArm)>0.01 % 不相等
    isSend=1;
    lastArm=arm;
end

== matlab function pixhawk_slib_sensors_actuators/TorqueThrust4Ctrls/ArmTrig ==
  data: u input; arm output; isSend output
function [arm,isSend] = fcn(u)

persistent lastArm;
if isempty(lastArm)
    lastArm=0;
end

isSend=0;
arm=u;

if abs(arm-lastArm)>0.01 % 不相等
    isSend=1;
    lastArm=arm;
end
